simulink library "Control_System_Library"  (Simulink 8.0)
settings: Solver=ode45  StartTime=0.0  StopTime=10.0  RelTol=1e-3
values from neighbouring files (symbols this model uses):
  B_bias = [0 0 0]    [Initialize_UKF_Function.m]
  B_Init_Inertial = wrldmagm(Alt, Lat, Long, 2013)*1E-9    [Initialize_UKF_Function.m]
  I_c = [3.4 3.4 1.9]    [Initialize_UKF_Function.m]    (also in UKF_quaternion_withBias.m)
  NED_Init = dcmecef2ned(Lat, Long)*ECEF_Init    [Initialize_UKF_Function.m]
  q_i_s0 = init_attitude    [Initialize_UKF_Function.m]
  q_s_c = [1 0 0 0]    [Initialize_UKF_Function.m]    (also in Satellite2Controller_Conversion.m = dcm2quat(R); UKF_quaternion_withBias.m = [1; 0; 0; 0])
  Time_Start = 0    [Initialize_UKF_Function.m]
  Ts = .1    (= 0.1)    [Initialize_UKF_Function.m]
  w_bias = 0*[0.5 0.2 0.15]    [Initialize_UKF_Function.m]    (also in UKF_quaternion_withBias.m = zeros(3,1))
  w_init_s = [rand_w_x rand_w_y rand_w_z]    [Initialize_UKF_Function.m]
undefined symbols (not defined in the file or in its folder): aeroassertmsg, c, cd, DiscIntNeverNeededParam, dyear, Earth, epoch, fm, fn, k, maxdef, Newton, Raphson, sgp4, snorm, WGS84
libraries: commnoisgen2 x6, aerolibconvert2 x4, simulink x3, aerolibutil x2, aerolibtransform2 x2, dspmtrx3 x1, aerolibgravitysys x1
(part 1 of 3)
settings Model: Creator=bajackso  LastModifiedBy=nwford

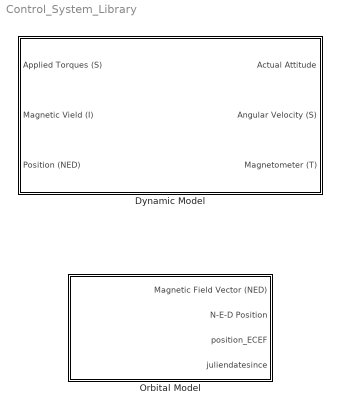
== system Control_System_Library ==
  Dynamic Model : Subsystem
  Orbital Model : Subsystem

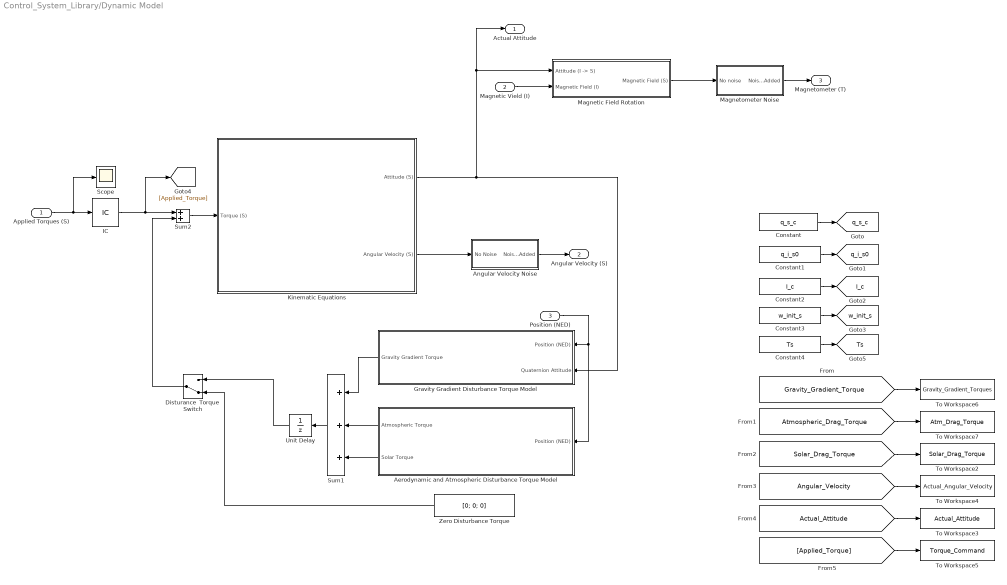
== system Control_System_Library/Dynamic Model ==
  Applied Torques (S) : Inport
  Magnetic Vield (I) : Inport  Port=2
  Position (NED) : Inport  Port=3
  Aerodynamic and Atmospheric Disturbance Torque Model : Subsystem
  Angular Velocity Noise : Subsystem
  Constant : Constant  Value=q_s_c
  Constant1 : Constant  Value=q_i_s0
  Constant2 : Constant  Value=I_c
  Constant3 : Constant  Value=w_init_s
  Constant4 : Constant  Value=Ts
  Disturance  Torque Switch : ManualSwitch  CurrentSetting=0
  Gravity Gradient Disturbance Torque Model : Subsystem
  IC : InitialCondition  Value=[0 0 0]
  Kinematic Equations : Subsystem
  Magnetic Field Rotation : Subsystem
  Magnetometer Noise : Subsystem
  Scope : Scope
      settings: TimeRange=10000
  Sum1 : Sum  Inputs=+++
  Sum2 : Sum
  To Workspace2 : ToWorkspace  VariableName=Solar_Drag_Torque  SampleTime=-1
      settings: Decimation=Decimation
  To Workspace3 : ToWorkspace  VariableName=Actual_Attitude  SampleTime=-1
      settings: Decimation=Decimation
  To Workspace4 : ToWorkspace  VariableName=Actual_Angular_Velocity  SampleTime=-1
      settings: Decimation=Decimation
  To Workspace5 : ToWorkspace  VariableName=Torque_Command  SampleTime=-1
      settings: Decimation=Decimation
  To Workspace6 : ToWorkspace  VariableName=Gravity_Gradient_Torques  SampleTime=-1
      settings: Decimation=Decimation
  To Workspace7 : ToWorkspace  VariableName=Atm_Drag_Torque  SampleTime=-1
      settings: Decimation=Decimation
  Unit Delay : UnitDelay  SampleTime=-1
  Zero Disturbance Torque : Constant  Value=[0; 0; 0]
  Actual Attitude : Outport
  Angular Velocity (S) : Outport  Port=2
  Magnetometer (T) : Outport  Port=3
  tag scope: I_c=global, Ts=global, q_i_s0=global, q_s_c=global, w_init_s=global
  wires:
  Unit Delay/1 -> Disturance  Torque Switch/1
  IC/1 -> [Applied_Torque], Sum2/1
  Kinematic Equations/1(Attitude (S)) -> Actual Attitude/1, Magnetic Field Rotation/1("Attitude (I -> S)"), Gravity Gradient Disturbance Torque Model/2(Quaternion Attitude)
  Applied Torques (S)/1 -> IC/1, Scope/1
  Sum2/1 -> Kinematic Equations/1(Torque (S))
  Sum1/1 -> Unit Delay/1
  Disturance  Torque Switch/1 -> Sum2/2
  Zero Disturbance Torque/1 -> Disturance  Torque Switch/2
  Position (NED)/1 -> Gravity Gradient Disturbance Torque Model/1(Position (NED)), Aerodynamic and Atmospheric Disturbance Torque Model/1(Position (NED))
  Gravity Gradient Disturbance Torque Model/1(Gravity Gradient Torque) -> Sum1/1
  Aerodynamic and Atmospheric Disturbance Torque Model/1(Atmospheric Torque) -> Sum1/2
  Aerodynamic and Atmospheric Disturbance Torque Model/2(Solar Torque) -> Sum1/3
  Angular Velocity Noise/1(Noise Added) -> Angular Velocity (S)/1
  Magnetometer Noise/1("Noise Added ") -> Magnetometer (T)/1
  Constant/1 -> [q_s_c]
  Constant1/1 -> [q_i_s0]
  Constant2/1 -> [I_c]
  Constant3/1 -> [w_init_s]
  Kinematic Equations/2(Angular Velocity (S)) -> Angular Velocity Noise/1(No Noise)
  Magnetic Vield (I)/1 -> Magnetic Field Rotation/2(Magnetic Field (I))
  Magnetic Field Rotation/1(Magnetic Field (S)) -> Magnetometer Noise/1(No noise)
  [Gravity_Gradient_Torque] -> To Workspace6/1
  [Atmospheric_Drag_Torque] -> To Workspace7/1
  [Solar_Drag_Torque] -> To Workspace2/1
  [Angular_Velocity] -> To Workspace4/1
  [Actual_Attitude] -> To Workspace3/1
  [Applied_Torque] -> To Workspace5/1
  Constant4/1 -> [Ts]

== system Control_System_Library/Orbital Model ==
  Constant : Constant  Value=Time_Start
  Digital Clock1 : DigitalClock  SampleTime=.1
  "JDepochdate " : Constant  Value=2456507.01579
  Rate Transition : RateTransition  X0=NED_Init
  Rate Transition1 : RateTransition  X0=B_Init_Inertial
  S2M : Gain  Gain=1/60
  SGP4 : MATLABFcn  MATLABFcn=sgp4(u(1))
  Subsystem : Subsystem
  Sum : Sum  Inputs=|++
  Sum1 : Sum  Inputs=|++
  gain : Gain  Gain=1/(60*24)
  km to m : Gain  Gain=1000
  Magnetic Field Vector (NED) : Outport  PortDimensions=3
  N-E-D Position : Outport  Port=2  PortDimensions=3
  position_ECEF : Outport  Port=3
  "juliendatesince " : Outport  Port=4  PortDimensions=1
  wires:
  Digital Clock1/1 -> S2M/1
  Subsystem/2(Position  (NED)) -> Rate Transition/1
  km to m/1 -> position_ECEF/1, Subsystem/1(Position  (ECEF))
  Subsystem/1(Magnetic Field  (NED)) -> Rate Transition1/1
  SGP4/1 -> km to m/1
  Rate Transition/1 -> N-E-D Position/1
  Rate Transition1/1 -> Magnetic Field Vector (NED)/1
  S2M/1 -> Sum/1
  Constant/1 -> Sum/2
  Sum/1 -> gain/1, SGP4/1
  "JDepochdate "/1 -> Sum1/1
  Sum1/1 -> "juliendatesince "/1
  gain/1 -> Sum1/2

== system Control_System_Library/Dynamic Model/Aerodynamic and Atmospheric Disturbance Torque Model ==
  Position (NED) : Inport
  MATLAB Function : MATLAB Function  TreatAsAtomicUnit=on
  MATLAB Function1 : MATLAB Function  TreatAsAtomicUnit=on
  Atmospheric Torque : Outport
  Solar Torque : Outport  Port=2
  tag scope: Atmospheric_Drag_Torque=global, Solar_Drag_Torque=global
  wires:
  MATLAB Function/1(ATM_Torque) -> [Atmospheric_Drag_Torque], Atmospheric Torque/1
  Position (NED)/1 -> MATLAB Function/1(R)
  MATLAB Function1/1(Solar_Torque) -> [Solar_Drag_Torque], Solar Torque/1

== system Control_System_Library/Dynamic Model/Angular Velocity Noise ==
  No Noise : Inport
  Manual Switch : ManualSwitch  CurrentSetting=0
  Mux : Mux  Inputs=3
  Sum : Sum  Inputs=|++
  X : commnoisgen2/Gaussian Noise Generator  m=w_bias(1)  d=gyro_noise  s=41  Ts=Ts  frameBased=off  sampPerFrame=1  orient=off  outDataType=double
  Y : commnoisgen2/Gaussian Noise Generator  m=w_bias(2)  d=gyro_noise  s=1235123  Ts=Ts  frameBased=off  sampPerFrame=1  orient=off  outDataType=double
  Z : commnoisgen2/Gaussian Noise Generator  m=w_bias(3)  d=gyro_noise  s=23523  Ts=Ts  frameBased=off  sampPerFrame=1  orient=off  outDataType=double
  Zero Noise : Constant  Value=0
  Noise Added : Outport
  wires:
  X/1 -> Mux/1
  Y/1 -> Mux/2
  Z/1 -> Mux/3
  No Noise/1 -> Sum/1
  Zero Noise/1 -> Manual Switch/2
  Mux/1 -> Manual Switch/1
  Sum/1 -> Noise Added/1
  Manual Switch/1 -> Sum/2

== system Control_System_Library/Dynamic Model/Gravity Gradient Disturbance Torque Model ==
  Position (NED) : Inport
  Quaternion Attitude : Inport  Port=2
  Conversion to Satellite Body Frame : aerolibutil/Quaternion Rotation
  MATLAB Function : MATLAB Function  TreatAsAtomicUnit=on
  Gravity Gradient Torque : Outport
  tag scope: Gravity_Gradient_Torque=global
  wires:
  MATLAB Function/1(G_grav) -> [Gravity_Gradient_Torque], Gravity Gradient Torque/1
  Quaternion Attitude/1 -> Conversion to Satellite Body Frame/1
  Position (NED)/1 -> Conversion to Satellite Body Frame/2
  Conversion to Satellite Body Frame/1 -> MATLAB Function/1(R)

== system Control_System_Library/Dynamic Model/Kinematic Equations ==
  Torque (S) : Inport
  Discrete-Time Integrator : DiscreteIntegrator  Commented=on  InitialConditionSource=external  InitialCondition=[0; 0; 0]  SampleTime=-1  ICPrevOutput=DiscIntNeverNeededParam  ICPrevScaledInput=DiscIntNeverNeededParam
  Discrete-Time Integrator1 : DiscreteIntegrator  Commented=on  InitialCondition=[0; 0; 0]  SampleTime=-1  ICPrevOutput=DiscIntNeverNeededParam  ICPrevScaledInput=DiscIntNeverNeededParam
  MATLAB Function : MATLAB Function  Commented=on  TreatAsAtomicUnit=on
  MATLAB Function1 : MATLAB Function  Commented=on  TreatAsAtomicUnit=on
  MATLAB Function2 : MATLAB Function  TreatAsAtomicUnit=on
  Matrix Multiply : Product  Commented=on  Multiplication=Matrix(*)
  Attitude (S) : Outport
  Angular Velocity (S) : Outport  Port=2
  tag scope: Actual_Attitude=global, Angular_Velocity=global
  wires:
  Discrete-Time Integrator/1 -> Matrix Multiply/2, MATLAB Function/3(w)
  MATLAB Function/1(w_dot) -> Discrete-Time Integrator/1
  Matrix Multiply/1 -> Discrete-Time Integrator1/1
  Discrete-Time Integrator1/1 -> MATLAB Function1/1(EA)
  MATLAB Function1/1(B) -> Matrix Multiply/1
  Torque (S)/1 -> MATLAB Function2/3(Torque_s)
  [I_c] -> MATLAB Function2/1(I_c)
  [q_i_s0] -> MATLAB Function2/4(q0_i_s)
  MATLAB Function2/1(w_s) -> [Angular_Velocity], Angular Velocity (S)/1
  MATLAB Function2/2(q_i_s) -> [Actual_Attitude], Attitude (S)/1
  [w_init_s] -> MATLAB Function2/2(w_init_s)
  [q_s_c] -> MATLAB Function2/5(q_s_c)
  [Ts] -> MATLAB Function2/6(Ts)

== system Control_System_Library/Dynamic Model/Magnetic Field Rotation ==
  "Attitude (I -> S)" : Inport
  Magnetic Field (I) : Inport  Port=2
  IC : InitialCondition  Value=q_i_s0
  IC1 : InitialCondition  Value=B_Init_Inertial
  Quaternion Rotation1 : aerolibutil/Quaternion Rotation
  Transpose1 : dspmtrx3/Transpose  Hermitian=off  overflowFlag=off
  Magnetic Field (S) : Outport
  wires:
  Quaternion Rotation1/1 -> Magnetic Field (S)/1
  Magnetic Field (I)/1 -> IC1/1
  Transpose1/1 -> Quaternion Rotation1/1
  "Attitude (I -> S)"/1 -> IC/1
  IC/1 -> Transpose1/1
  IC1/1 -> Quaternion Rotation1/2

== system Control_System_Library/Dynamic Model/Magnetometer Noise ==
  No noise : Inport
  Manual Switch : ManualSwitch
  Mux : Mux  Inputs=3
  Sum : Sum  Inputs=|++
  X : commnoisgen2/Gaussian Noise Generator  m=B_bias(1)  d=B_noise  s=2341  Ts=Ts  frameBased=off  sampPerFrame=1  orient=off  outDataType=double
  Y : commnoisgen2/Gaussian Noise Generator  m=B_bias(2)  d=B_noise  s=64236  Ts=Ts  frameBased=off  sampPerFrame=1  orient=off  outDataType=double
  Z : commnoisgen2/Gaussian Noise Generator  m=B_bias(3)  d=B_noise  s=346312  Ts=Ts  frameBased=off  sampPerFrame=1  orient=off  outDataType=double
  Zero Noise : Constant  Value=0
  "Noise Added " : Outport
  wires:
  X/1 -> Mux/1
  Y/1 -> Mux/2
  Z/1 -> Mux/3
  Mux/1 -> Manual Switch/1
  Zero Noise/1 -> Manual Switch/2
  Manual Switch/1 -> Sum/2
  No noise/1 -> Sum/1
  Sum/1 -> "Noise Added "/1

== system Control_System_Library/Orbital Model/Subsystem ==
  Position  (ECEF) : Inport
  Demux : Demux  Outputs=2
  Direction Cosine Matrix ECEF to NED : aerolibtransform2/Direction Cosine Matrix ECEF to NED
  ECEF Position to LLA1 : aerolibtransform2/ECEF Position to LLA  units=Metric (MKS)  ptype=Earth (WGS84)  F=1/298.257223563  R=6378137
  Gain : Gain  Gain=1E-9
  Matrix Multiply : Product  Multiplication=Matrix(*)
  World Magnetic Model 2010 : Subsystem  AncestorBlock=aerolibgravity2/World Magnetic Model 2010  mask(World Magnetic Model 2010){units=Metric (MKS), time_in=off, month=January, day=1, year=2010, action=Error, h_out=off, dec_out=off, inc_out=off, ti_out=off}
      mask prompts: time_in "Input decimal year"; action "Action for out of range input:"; h_out "Output horizontal intensity"; dec_out "Output declination"; inc_out "Output inclination"; ti_out "Output total intensity"
      mask help:
      | Calculate the Earth's magnetic field at a specific location and time using the World Magnetic Model (WMM). This model is valid for the year 2010 through the year 2015.
      |
      | The WMM-2010 can be found on the web at http://www.ngdc.noaa.gov/geomag/WMM/DoDWMM.shtml and in "NOAA Technical Report: The US/UK World Magnetic Model for 2010-2015 ".
      |
      | Height is entered in length units of selected unit system. Latitude and longitude are entered in degrees.
      mask init:
      | [ports,dyear,maxdef,epoch,c,cd,fn,fm,snorm,k]=aeroicon('aeroblkwmm2010','icon');
      mask Help: eval('asbhelp');
      mask TypeOptions units: Metric (MKS) | English
      mask Callback time_in: aeroicon('aeroblkwmm');
      mask TypeOptions month: January | February | March | April | May | June | July | August | September | October | November | December
      mask Callback month: aeroicon('aeroblkwmm');
      mask TypeOptions day: 1 | 2 | 3 | 4 | 5 | 6 | 7 | 8 | 9 | 10 | 11 | 12 | 13 | 14 | 15 | 16 | 17 | 18 | 19 | 20 | 21 | 22 | 23 | 24 | 25 | 26 | 27 | 28 | 29 | 30 | 31
      mask Callback day: aeroicon('aeroblkwmm');
      mask TypeOptions year: 2010 | 2011 | 2012 | 2013 | 2014 | 2015
      mask Callback year: aeroicon('aeroblkwmm');
      mask TypeOptions action: None | Warning | Error
      mask Display:
      | port_label(ports(1).type,ports(1).port,ports(1).txt);
      | port_label(ports(2).type,ports(2).port,ports(2).txt,'texmode','on');
      | port_label(ports(3).type,ports(3).port,ports(3).txt,'texmode','on');
      | port_label(ports(4).type,ports(4).port,ports(4).txt);
      | port_label(ports(5).type,ports(5).port,ports(5).txt);
      | port_label(ports(6).type,ports(6).port,ports(6).txt);
      | port_label(ports(7).type,ports(7).port,ports(7).txt);
      | port_label(ports(8).type,ports(8).port,ports(8).txt);
      | port_label(ports(9).type,ports(9).port,ports(9).txt);
  Magnetic Field  (NED) : Outport
  Position  (NED) : Outport  Port=2
  wires:
  World Magnetic Model 2010/1(Magnetic Field) -> Gain/1
  Gain/1 -> Magnetic Field  (NED)/1
  Position  (ECEF)/1 -> ECEF Position to LLA1/1, Matrix Multiply/2
  ECEF Position to LLA1/2 -> World Magnetic Model 2010/1(Altitude)
  Demux/1 -> World Magnetic Model 2010/2(Latitude)
  Demux/2 -> World Magnetic Model 2010/3(Longitude)
  ECEF Position to LLA1/1 -> Demux/1, Direction Cosine Matrix ECEF to NED/1
  Direction Cosine Matrix ECEF to NED/1 -> Matrix Multiply/1
  Matrix Multiply/1 -> Position  (NED)/1

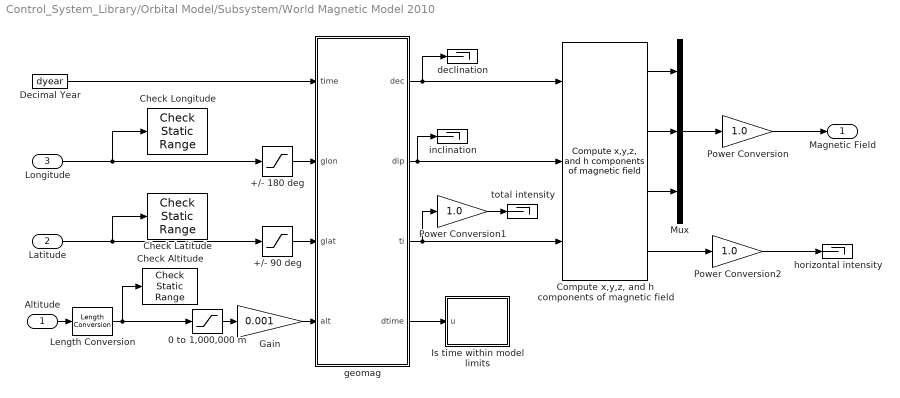
== system Control_System_Library/Orbital Model/Subsystem/World Magnetic Model 2010 ==
  Altitude : Inport
  Latitude : Inport  Port=2
  Longitude : Inport  Port=3
  +/- 180 deg : Saturate  UpperLimit=180.0  LowerLimit=-180.0
  +/- 90 deg : Saturate  UpperLimit=90.0  LowerLimit=-90.0
  0 to 1,000,000 m : Saturate  UpperLimit=1000000.0  LowerLimit=0
  Check Altitude : simulink/Model Verification/Check  Static Range  Description=0 <= u <= 1000000  max=1000000  max_included=on  min=0  min_included=on  enabled=on  callback=aeroassertmsg('aeroblkwmm','alt','error')  stopWhenAssertionFail=on  export=off  icon=graphic
  Check Latitude : simulink/Model Verification/Check  Static Range  Description=-90 <= u <= 90  max=90  max_included=on  min=-90  min_included=on  enabled=on  callback=aeroassertmsg('aeroblkwmm','lat','error')  stopWhenAssertionFail=on  export=off  icon=graphic
  Check Longitude : simulink/Model Verification/Check  Static Range  Description=-180 <= u <= 180  max=180  max_included=on  min=-180  min_included=on  enabled=on  callback=aeroassertmsg('aeroblkwmm','lon','error')  stopWhenAssertionFail=on  export=off  icon=graphic
  "Compute x,y,z, and h components of magnetic field" : aerolibgravitysys/Compute x,y,z, and h components of magnetic field
  Decimal Year : Constant  Value=dyear  OutDataTypeStr=Inherit: Inherit via back propagation
  Gain : Gain  Gain=0.001  SaturateOnIntegerOverflow=on  OutDataTypeStr=Inherit: Same as input  ParamDataTypeStr=Inherit: Same as input
  Is time within model limits : Subsystem  Description=0 <= u <= 5  mask(Checks_SRange){max=5, max_included=on, min=0, min_included=on, enabled=on, callback=aeroassertmsg('aeroblkwmm','time','error'), stopWhenAssertionFail=on, export=off, icon=graphic}
      mask prompts: max "Upper bound:"; max_included "Inclusive upper bound"; min "Lower bound:"; min_included "Inclusive lower bound"; enabled "Enable assertion"; callback "Simulation callback when assertion fails (optional):"; stopWhenAssertionFail "Stop simulation when assertion fails"; export "Output assertion signal"; icon "Select icon type:"
      mask help: Assert that the input signal lies between a static lower and upper bound or optionally equals either bound.
      mask init:
      | update_assert_sys(gcbh);
      mask TypeOptions icon: graphic | text
      mask Display: image(imread('Checks_SRange.bmp','bmp'),'center')
  Length Conversion : aerolibconvert2/Length Conversion  IU=m  OU=m
  Mux : Mux  Inputs=3
  Power Conversion : Gain  Gain=1.0  SaturateOnIntegerOverflow=on  OutDataTypeStr=Inherit: Same as input  ParamDataTypeStr=Inherit: Same as input
  Power Conversion1 : Gain  Gain=1.0  SaturateOnIntegerOverflow=on  OutDataTypeStr=Inherit: Same as input  ParamDataTypeStr=Inherit: Same as input
  Power Conversion2 : Gain  Gain=1.0  SaturateOnIntegerOverflow=on  OutDataTypeStr=Inherit: Same as input  ParamDataTypeStr=Inherit: Same as input
  declination : Terminator
  geomag : Subsystem  AncestorBlock=aerolibgravitysys/geomag
  horizontal intensity : Terminator
  inclination : Terminator
  total intensity : Terminator
  Magnetic Field : Outport
  wires:
  geomag/4(dtime) -> Is time within model limits/1(u)
  0 to 1,000,000 m/1 -> Gain/1
  +/- 180 deg/1 -> geomag/2(glon)
  +/- 90 deg/1 -> geomag/3(glat)
  Power Conversion2/1 -> horizontal intensity/1
  Power Conversion1/1 -> total intensity/1
  Power Conversion/1 -> Magnetic Field/1
  Mux/1 -> Power Conversion/1
  geomag/1(dec) -> declination/1, "Compute x,y,z, and h components of magnetic field"/1
  Gain/1 -> geomag/4(alt)
  Longitude/1 -> Check Longitude/1, +/- 180 deg/1
  Latitude/1 -> Check Latitude/1, +/- 90 deg/1
  geomag/3(ti) -> Power Conversion1/1, "Compute x,y,z, and h components of magnetic field"/3
  geomag/2(dip) -> inclination/1, "Compute x,y,z, and h components of magnetic field"/2
  Decimal Year/1 -> geomag/1(time)
  "Compute x,y,z, and h components of magnetic field"/4 -> Power Conversion2/1
  "Compute x,y,z, and h components of magnetic field"/3 -> Mux/3
  "Compute x,y,z, and h components of magnetic field"/2 -> Mux/2
  "Compute x,y,z, and h components of magnetic field"/1 -> Mux/1
  Length Conversion/1 -> Check Altitude/1, 0 to 1,000,000 m/1
  Altitude/1 -> Length Conversion/1

== system Control_System_Library/Orbital Model/Subsystem/World Magnetic Model 2010/Is time within model limits ==
  u : Inport
  Assertion : Assertion  Enabled=on  AssertionFailFcn=evalin('base',callback)
  conjunction : Logic
  max_relop : RelationalOperator  Operator=<=  InputSameDT=on
  max_val : Constant  Value=max
  maxtype : DataTypeConversion  SaturateOnIntegerOverflow=on  RndMeth=Zero
  min_relop : RelationalOperator  Operator=<=  InputSameDT=on
  min_val : Constant  Value=min
  mintype : DataTypeConversion  SaturateOnIntegerOverflow=on  RndMeth=Zero
  out : Terminator
  wires:
  u/1 -> min_relop/2, max_relop/1
  min_val/1 -> mintype/1
  max_val/1 -> maxtype/1
  min_relop/1 -> conjunction/1
  max_relop/1 -> conjunction/2
  conjunction/1 -> out/1, Assertion/1
  mintype/1 -> min_relop/1
  maxtype/1 -> max_relop/2

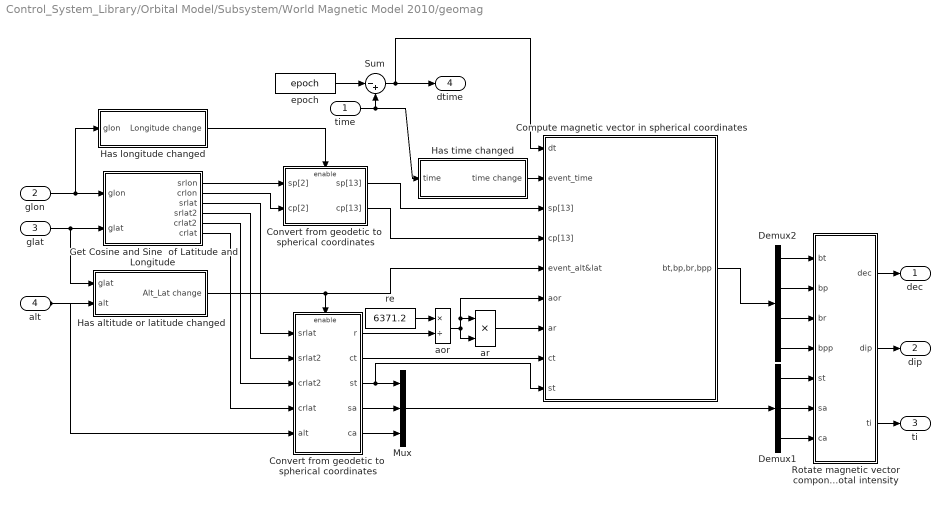
== system Control_System_Library/Orbital Model/Subsystem/World Magnetic Model 2010/geomag ==
  time : Inport
  glon : Inport  Port=2
  glat : Inport  Port=3
  alt : Inport  Port=4
  Compute magnetic vector in spherical coordinates : Subsystem  TreatAsAtomicUnit=on
  Convert from geodetic to  spherical coordinates : Subsystem  TreatAsAtomicUnit=on
  "Convert from geodetic to  spherical coordinates " : Subsystem
  Demux1 : Demux  Outputs=3
  Demux2 : Demux
  Get Cosine and Sine  of Latitude and Longitude : Subsystem
  Has altitude or latitude changed : Subsystem
  "Has longitude changed " : Subsystem
  Has time changed : Subsystem
  Mux : Mux  Inputs=3
  "Rotate magnetic vector components  to geodetic from spherical and  compute declination, inclination  and total intensity" : Subsystem
  Sum : Sum  Inputs=|-+  SaturateOnIntegerOverflow=on
  aor : Product  Inputs=*/  SaturateOnIntegerOverflow=on  OutDataTypeStr=Inherit: Same as first input
  ar : Product  SaturateOnIntegerOverflow=on  OutDataTypeStr=Inherit: Same as first input
  epoch : Constant  Value=epoch  OutDataTypeStr=Inherit: Inherit via back propagation
  re : Constant  Value=6371.2  OutDataTypeStr=Inherit: Inherit via back propagation
  dec : Outport
  dip : Outport  Port=2
  ti : Outport  Port=3
  dtime : Outport  Port=4
  wires:
  Demux2/3 -> "Rotate magnetic vector components  to geodetic from spherical and  compute declination, inclination  and total intensity"/3(br)
  Demux2/2 -> "Rotate magnetic vector components  to geodetic from spherical and  compute declination, inclination  and total intensity"/2(bp)
  Compute magnetic vector in spherical coordinates/1(bt,bp,br,bpp) -> Demux2/1
  Demux1/3 -> "Rotate magnetic vector components  to geodetic from spherical and  compute declination, inclination  and total intensity"/7(ca)
  Demux1/2 -> "Rotate magnetic vector components  to geodetic from spherical and  compute declination, inclination  and total intensity"/6(sa)
  Demux1/1 -> "Rotate magnetic vector components  to geodetic from spherical and  compute declination, inclination  and total intensity"/5(st)
  Demux2/4 -> "Rotate magnetic vector components  to geodetic from spherical and  compute declination, inclination  and total intensity"/4(bpp)
  Demux2/1 -> "Rotate magnetic vector components  to geodetic from spherical and  compute declination, inclination  and total intensity"/1(bt)
  Mux/1 -> Demux1/1
  Convert from geodetic to  spherical coordinates/5(ca) -> Mux/3
  Convert from geodetic to  spherical coordinates/4(sa) -> Mux/2
  Convert from geodetic to  spherical coordinates/3(st) -> Compute magnetic vector in spherical coordinates/9(st), Mux/1
  epoch/1 -> Sum/1
  Convert from geodetic to  spherical coordinates/2(ct) -> Compute magnetic vector in spherical coordinates/8(ct)
  Get Cosine and Sine  of Latitude and Longitude/6(crlat) -> Convert from geodetic to  spherical coordinates/4(crlat)
  Get Cosine and Sine  of Latitude and Longitude/3(srlat) -> Convert from geodetic to  spherical coordinates/1(srlat)
  "Rotate magnetic vector components  to geodetic from spherical and  compute declination, inclination  and total intensity"/3(ti) -> ti/1
  "Rotate magnetic vector components  to geodetic from spherical and  compute declination, inclination  and total intensity"/2(dip) -> dip/1
  "Rotate magnetic vector components  to geodetic from spherical and  compute declination, inclination  and total intensity"/1(dec) -> dec/1
  ar/1 -> Compute magnetic vector in spherical coordinates/7(ar)
  re/1 -> aor/1
  Convert from geodetic to  spherical coordinates/1(r) -> aor/2
  aor/1 -> ar/1, Compute magnetic vector in spherical coordinates/6(aor), ar/2
  "Convert from geodetic to  spherical coordinates "/2(cp[13]) -> Compute magnetic vector in spherical coordinates/4(cp[13])
  "Convert from geodetic to  spherical coordinates "/1(sp[13]) -> Compute magnetic vector in spherical coordinates/3(sp[13])
  Has altitude or latitude changed/1(Alt_Lat change) -> Compute magnetic vector in spherical coordinates/5(event_alt&lat), Convert from geodetic to  spherical coordinates/Enable
  Get Cosine and Sine  of Latitude and Longitude/5(crlat2) -> Convert from geodetic to  spherical coordinates/3(crlat2)
  Get Cosine and Sine  of Latitude and Longitude/4(srlat2) -> Convert from geodetic to  spherical coordinates/2(srlat2)
  Get Cosine and Sine  of Latitude and Longitude/2(crlon) -> "Convert from geodetic to  spherical coordinates "/2(cp[2])
  Get Cosine and Sine  of Latitude and Longitude/1(srlon) -> "Convert from geodetic to  spherical coordinates "/1(sp[2])
  alt/1 -> Convert from geodetic to  spherical coordinates/5(alt), Has altitude or latitude changed/2(alt)
  glat/1 -> Get Cosine and Sine  of Latitude and Longitude/2(glat), Has altitude or latitude changed/1(glat)
  glon/1 -> Get Cosine and Sine  of Latitude and Longitude/1(glon), "Has longitude changed "/1(glon)
  "Has longitude changed "/1(Longitude change) -> "Convert from geodetic to  spherical coordinates "/Enable
  Has time changed/1(time change) -> Compute magnetic vector in spherical coordinates/2(event_time)
  time/1 -> Sum/2, Has time changed/1(time)
  Sum/1 -> dtime/1, Compute magnetic vector in spherical coordinates/1(dt)

== system Control_System_Library/Orbital Model/Subsystem/World Magnetic Model 2010/geomag/Compute magnetic vector in spherical coordinates ==
  dt : Inport
  event_time : Inport  Port=2
  sp[13] : Inport  Port=3
  cp[13] : Inport  Port=4
  event_alt&lat : Inport  Port=5
  aor : Inport  Port=6
  ar : Inport  Port=7
  ct : Inport  Port=8
  st : Inport  Port=9
  Constant : Constant  OutDataTypeStr=Inherit: Inherit via back propagation
  For Iterator : ForIterator  ResetStates=reset  IterationLimit=maxdef
  For Iterator Subsystem : Subsystem  TreatAsAtomicUnit=on
  Mux : Mux
  Product8 : Product  SaturateOnIntegerOverflow=on  OutDataTypeStr=Inherit: Same as first input
  Sum : Sum  Inputs=++|  SaturateOnIntegerOverflow=on
  Sum1 : Sum  Inputs=++|  SaturateOnIntegerOverflow=on
  Unit Delay : UnitDelay  SampleTime=-1
  Unit Delay2 : UnitDelay  InitialCondition=[0 0 0 0]  SampleTime=-1
  ar(n) : Switch  Criteria=u2 > Threshold  Threshold=1  SaturateOnIntegerOverflow=on
  bt,bp,br,bpp : Outport
  wires:
  Sum1/1 -> Unit Delay2/1, bt,bp,br,bpp/1
  Unit Delay2/1 -> Sum1/1
  Mux/1 -> Sum1/2
  For Iterator Subsystem/4(bpp) -> Mux/4
  For Iterator Subsystem/3(br) -> Mux/3
  For Iterator Subsystem/2(bp) -> Mux/2
  For Iterator Subsystem/1(bt) -> Mux/1
  dt/1 -> For Iterator Subsystem/10(dt)
  cp[13]/1 -> For Iterator Subsystem/9(cp)
  sp[13]/1 -> For Iterator Subsystem/8(sp)
  st/1 -> For Iterator Subsystem/7(st)
  ct/1 -> For Iterator Subsystem/6(ct)
  Constant/1 -> Sum/2
  Sum/1 -> For Iterator Subsystem/3(D4)
  ar(n)/1 -> Product8/1
  Product8/1 -> For Iterator Subsystem/1(ar), Unit Delay/1
  Unit Delay/1 -> ar(n)/1
  aor/1 -> Product8/2
  event_time/1 -> For Iterator Subsystem/5(event_time)
  ar/1 -> ar(n)/3
  event_alt&lat/1 -> For Iterator Subsystem/4(event_alt&lat)
  For Iterator/1 -> Sum/1, For Iterator Subsystem/2(n), ar(n)/2

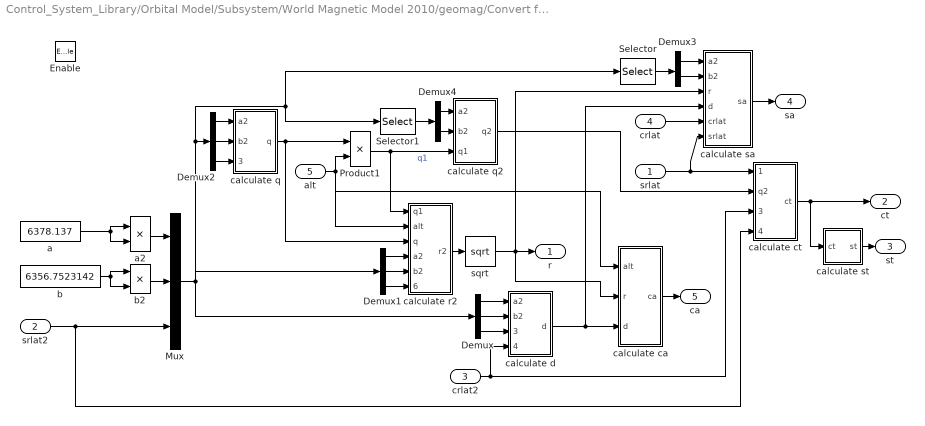
== system Control_System_Library/Orbital Model/Subsystem/World Magnetic Model 2010/geomag/Convert from geodetic to  spherical coordinates ==
  srlat : Inport
  srlat2 : Inport  Port=2
  crlat2 : Inport  Port=3
  crlat : Inport  Port=4
  alt : Inport  Port=5
  Enable : EnablePort  PropagateVarSize=During execution
  Demux : Demux  Outputs=3
  Demux1 : Demux  Outputs=3
  Demux2 : Demux  Outputs=3
  Demux3 : Demux  Outputs=2
  Demux4 : Demux  Outputs=2
  Mux : Mux  Inputs=3
  Product1 : Product  SaturateOnIntegerOverflow=on  OutDataTypeStr=Inherit: Same as first input
  Selector : Selector  InputPortWidth=3  IndexOptions=Index vector (dialog)  Indices=[1 2]  OutputSizes=1
  Selector1 : Selector  InputPortWidth=3  IndexOptions=Index vector (dialog)  Indices=[1 2]  OutputSizes=1
  a : Constant  Value=6378.137  OutDataTypeStr=Inherit: Inherit via back propagation
  a2 : Product  SaturateOnIntegerOverflow=on  OutDataTypeStr=Inherit: Same as first input
  b : Constant  Value=6356.7523142  OutDataTypeStr=Inherit: Inherit via back propagation
  b2 : Product  SaturateOnIntegerOverflow=on  OutDataTypeStr=Inherit: Same as first input
  calculate ca : Subsystem
  calculate ct : Subsystem
  calculate d : Subsystem
  calculate q : Subsystem
  calculate q2 : Subsystem
  calculate r2 : Subsystem
  calculate sa : Subsystem
  calculate st : Subsystem
  sqrt : Sqrt  AlgorithmType=Newton-Raphson  SaturateOnIntegerOverflow=on
  r : Outport
  ct : Outport  Port=2
  st : Outport  Port=3
  sa : Outport  Port=4
  ca : Outport  Port=5
  wires:
  Demux/3 -> calculate d/3(srlat2)
  Demux4/2 -> calculate q2/2(b2)
  Demux4/1 -> calculate q2/1(a2)
  Selector1/1 -> Demux4/1
  Selector/1 -> Demux3/1
  Demux3/2 -> calculate sa/2(b2)
  Demux3/1 -> calculate sa/1(a2)
  Mux/1 -> Selector/1, Selector1/1, Demux2/1, Demux/1, Demux1/1
  Demux2/3 -> calculate q/3(srlat2)
  Demux2/2 -> calculate q/2(b2)
  Demux2/1 -> calculate q/1(a2)
  Demux1/3 -> calculate r2/6(srlat2)
  Demux1/2 -> calculate r2/5(b2)
  Demux1/1 -> calculate r2/4(a2)
  Demux/1 -> calculate d/1(a2)
  Demux/2 -> calculate d/2(b2)
  calculate q2/1(q2) -> calculate ct/2(q2)
  b2/1 -> Mux/2
  b/1 -> b2/1, b2/2
  a2/1 -> Mux/1
  a/1 -> a2/1, a2/2
  calculate sa/1(sa) -> sa/1
  crlat/1 -> calculate sa/5(crlat)
  calculate ca/1(ca) -> ca/1
  calculate d/1(d) -> calculate sa/4(d), calculate ca/3(d)
  sqrt/1 -> calculate ca/2(r), calculate sa/3(r), r/1
  calculate r2/1(r2) -> sqrt/1
  calculate st/1(st) -> st/1
  calculate ct/1(ct) -> calculate st/1(ct), ct/1
  srlat/1 -> calculate sa/6(srlat), calculate ct/1(srlat)
  crlat2/1 -> calculate ct/3(crlat2), calculate d/4(crlat2)
  alt/1 -> calculate r2/2(alt), calculate ca/1(alt), Product1/2
  Product1/1 -> calculate r2/1(q1), calculate q2/3(q1)  "q1"
  calculate q/1(q) -> calculate r2/3(q), Product1/1
  srlat2/1 -> Mux/3, calculate ct/4(srlat2)

== system Control_System_Library/Orbital Model/Subsystem/World Magnetic Model 2010/geomag/Convert from geodetic to  spherical coordinates  ==
  sp[2] : Inport
  cp[2] : Inport  Port=2
  Enable : EnablePort  PropagateVarSize=During execution
  For Iterator Subsystem : Subsystem  TreatAsAtomicUnit=on
  Mux : Mux  Inputs=3
  Mux1 : Mux  Inputs=3
  cp[1] : Constant  OutDataTypeStr=Inherit: Inherit via back propagation
  sp[1] : Constant  Value=0  OutDataTypeStr=Inherit: Inherit via back propagation
  sp[13] : Outport  InitialOutput=[ zeros(1,13) ]
  cp[13] : Outport  Port=2  InitialOutput=[ zeros(1,13) ]
  wires:
  sp[1]/1 -> Mux1/1
  cp[1]/1 -> Mux/1
  Mux/1 -> cp[13]/1
  For Iterator Subsystem/2(cp[11]) -> Mux/3
  For Iterator Subsystem/1(sp[11]) -> Mux1/3
  cp[2]/1 -> For Iterator Subsystem/2(cp[2]), Mux/2
  sp[2]/1 -> For Iterator Subsystem/1(sp[2]), Mux1/2
  Mux1/1 -> sp[13]/1

== system Control_System_Library/Orbital Model/Subsystem/World Magnetic Model 2010/geomag/Get Cosine and Sine  of Latitude and Longitude ==
  glon : Inport
  glat : Inport  Port=2
  Angle Conversion : aerolibconvert2/Angle Conversion  IU=deg  OU=rad
  Demux : Demux  Outputs=2
  Demux1 : Demux  Outputs=2
  Mux : Mux  Inputs=2
  Product : Product  SaturateOnIntegerOverflow=on  OutDataTypeStr=Inherit: Same as first input
  Product1 : Product  SaturateOnIntegerOverflow=on  OutDataTypeStr=Inherit: Same as first input
  sincos : Trigonometry  Operator=sincos
  srlon : Outport
  crlon : Outport  Port=2
  srlat : Outport  Port=3
  srlat2 : Outport  Port=4
  crlat2 : Outport  Port=5
  crlat : Outport  Port=6
  wires:
  Demux1/2 -> Product1/2, Product1/1, crlat/1
  Demux/2 -> Product/2, Product/1, srlat/1
  Product1/1 -> crlat2/1
  Product/1 -> srlat2/1
  Demux1/1 -> crlon/1
  Demux/1 -> srlon/1
  glat/1 -> Mux/2
  glon/1 -> Mux/1
  sincos/2 -> Demux1/1
  sincos/1 -> Demux/1
  Mux/1 -> Angle Conversion/1
  Angle Conversion/1 -> sincos/1

== system Control_System_Library/Orbital Model/Subsystem/World Magnetic Model 2010/geomag/Has altitude or latitude changed ==
  glat : Inport
  alt : Inport  Port=2
  Logical Operator : Logic  Operator=OR  AllPortsSameDT=off
  Relational Operator : RelationalOperator  Operator=~=
  Relational Operator1 : RelationalOperator  Operator=~=
  oalt : Memory  X0=-1000  InheritSampleTime=on
  olat : Memory  X0=-1000  InheritSampleTime=on
  Alt_Lat change : Outport
  wires:
  Logical Operator/1 -> Alt_Lat change/1
  glat/1 -> olat/1, Relational Operator/1
  Relational Operator1/1 -> Logical Operator/2
  Relational Operator/1 -> Logical Operator/1
  oalt/1 -> Relational Operator1/2
  olat/1 -> Relational Operator/2
  alt/1 -> oalt/1, Relational Operator1/1

== system Control_System_Library/Orbital Model/Subsystem/World Magnetic Model 2010/geomag/Has longitude changed  ==
  glon : Inport
  Relational Operator : RelationalOperator  Operator=~=
  olon : Memory  X0=-1000  InheritSampleTime=on
  Longitude change : Outport
  wires:
  Relational Operator/1 -> Longitude change/1
  glon/1 -> olon/1, Relational Operator/1
  olon/1 -> Relational Operator/2

== system Control_System_Library/Orbital Model/Subsystem/World Magnetic Model 2010/geomag/Has time changed ==
  time : Inport
  Relational Operator : RelationalOperator  Operator=~=
  otime : Memory  X0=-1000  InheritSampleTime=on
  time change : Outport
  wires:
  otime/1 -> Relational Operator/2
  time/1 -> Relational Operator/1, otime/1
  Relational Operator/1 -> time change/1

== system Control_System_Library/Orbital Model/Subsystem/World Magnetic Model 2010/geomag/Rotate magnetic vector components  to geodetic from spherical and  compute declination, inclination  and total intensity ==
  bt : Inport
  bp : Inport  Port=2
  br : Inport  Port=3
  bpp : Inport  Port=4
  st : Inport  Port=5
  sa : Inport  Port=6
  ca : Inport  Port=7
  Calculate bx : Subsystem
  Calculate by : Subsystem
  Calculate bz : Subsystem
  "Compute declination, inclination,  and total intensity" : Subsystem
  Demux : Demux
  Demux1 : Demux
  Mux : Mux
  dec : Outport
  dip : Outport  Port=2
  ti : Outport  Port=3
  wires:
  "Compute declination, inclination,  and total intensity"/2(dip) -> dip/1
  "Compute declination, inclination,  and total intensity"/1(dec) -> dec/1
  Calculate bz/1(bz) -> "Compute declination, inclination,  and total intensity"/3(bz)
  Calculate bx/1(bx) -> "Compute declination, inclination,  and total intensity"/2(bx)
  Calculate by/1(by) -> "Compute declination, inclination,  and total intensity"/1(by)
  "Compute declination, inclination,  and total intensity"/3(ti) -> ti/1
  Demux1/4 -> Calculate bz/4(br)
  Demux1/3 -> Calculate bz/3(bt)
  Demux1/2 -> Calculate bz/2(sa)
  Demux1/1 -> Calculate bz/1(ca)
  Mux/1 -> Demux1/1, Demux/1
  Demux/4 -> Calculate bx/4(br)
  Demux/3 -> Calculate bx/3(bt)
  Demux/2 -> Calculate bx/2(sa)
  Demux/1 -> Calculate bx/1(ca)
  br/1 -> Mux/4
  bt/1 -> Mux/3
  sa/1 -> Mux/2
  ca/1 -> Mux/1
  bp/1 -> Calculate by/1(bp)
  bpp/1 -> Calculate by/3(bpp)
  st/1 -> Calculate by/2(st)

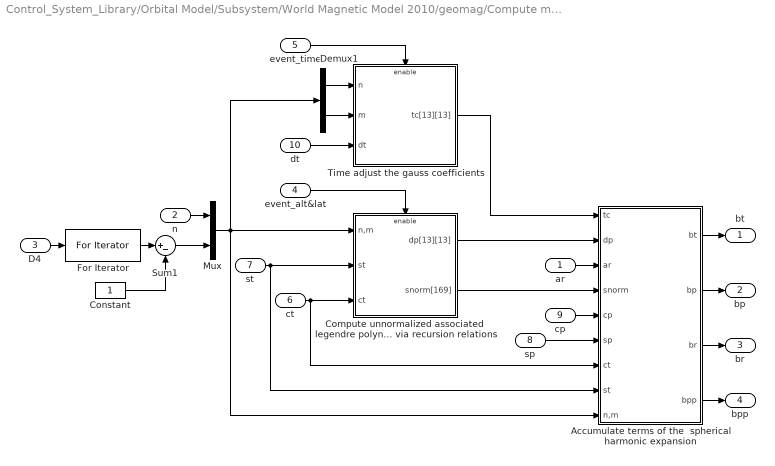
== system Control_System_Library/Orbital Model/Subsystem/World Magnetic Model 2010/geomag/Compute magnetic vector in spherical coordinates/For Iterator Subsystem ==
  ar : Inport
  n : Inport  Port=2
  D4 : Inport  Port=3
  event_alt&lat : Inport  Port=4
  event_time : Inport  Port=5
  ct : Inport  Port=6
  st : Inport  Port=7
  sp : Inport  Port=8
  cp : Inport  Port=9
  dt : Inport  Port=10
  Accumulate terms of the  spherical harmonic expansion : Subsystem
  Compute unnormalized associated  legendre polynomials and  derivatives via recursion relations : Subsystem  TreatAsAtomicUnit=on
  Constant : Constant  OutDataTypeStr=Inherit: Inherit via back propagation
  Demux1 : Demux  Outputs=2
  For Iterator : ForIterator  ResetStates=reset  IterationSource=external  IterationLimit=maxdef
  Mux : Mux  Inputs=2
  Sum1 : Sum  Inputs=|+-  SaturateOnIntegerOverflow=on  OutDataTypeStr=Inherit: Same as first input
  Time adjust the gauss coefficients : Subsystem  TreatAsAtomicUnit=on
  bt : Outport
  bp : Outport  Port=2
  br : Outport  Port=3
  bpp : Outport  Port=4
  wires:
  Accumulate terms of the  spherical harmonic expansion/4(bpp) -> bpp/1
  Sum1/1 -> Mux/2
  For Iterator/1 -> Sum1/1
  Demux1/2 -> Time adjust the gauss coefficients/2(m)
  Demux1/1 -> Time adjust the gauss coefficients/1(n)
  n/1 -> Mux/1
  Mux/1 -> Accumulate terms of the  spherical harmonic expansion/9(n,m), Compute unnormalized associated  legendre polynomials and  derivatives via recursion relations/1(n,m), Demux1/1
  Time adjust the gauss coefficients/1(tc[13][13]) -> Accumulate terms of the  spherical harmonic expansion/1(tc)
  ar/1 -> Accumulate terms of the  spherical harmonic expansion/3(ar)
  Accumulate terms of the  spherical harmonic expansion/2(bp) -> bp/1
  Accumulate terms of the  spherical harmonic expansion/1(bt) -> bt/1
  Accumulate terms of the  spherical harmonic expansion/3(br) -> br/1
  Compute unnormalized associated  legendre polynomials and  derivatives via recursion relations/1(dp[13][13]) -> Accumulate terms of the  spherical harmonic expansion/2(dp)
  Compute unnormalized associated  legendre polynomials and  derivatives via recursion relations/2(snorm[169]) -> Accumulate terms of the  spherical harmonic expansion/4(snorm)
  sp/1 -> Accumulate terms of the  spherical harmonic expansion/6(sp)
  cp/1 -> Accumulate terms of the  spherical harmonic expansion/5(cp)
  ct/1 -> Accumulate terms of the  spherical harmonic expansion/7(ct), Compute unnormalized associated  legendre polynomials and  derivatives via recursion relations/3(ct)
  st/1 -> Accumulate terms of the  spherical harmonic expansion/8(st), Compute unnormalized associated  legendre polynomials and  derivatives via recursion relations/2(st)
  dt/1 -> Time adjust the gauss coefficients/3(dt)
  event_time/1 -> Time adjust the gauss coefficients/Enable
  Constant/1 -> Sum1/2
  event_alt&lat/1 -> Compute unnormalized associated  legendre polynomials and  derivatives via recursion relations/Enable
  D4/1 -> For Iterator/1

== system Control_System_Library/Orbital Model/Subsystem/World Magnetic Model 2010/geomag/Convert from geodetic to  spherical coordinates/calculate ca ==
  alt : Inport
  r : Inport  Port=2
  d : Inport  Port=3
  Product11 : Product  Inputs=*/  SaturateOnIntegerOverflow=on  OutDataTypeStr=Inherit: Same as first input
  Sum8 : Sum  Inputs=|++  SaturateOnIntegerOverflow=on
  ca : Outport
  wires:
  Product11/1 -> ca/1
  d/1 -> Sum8/2
  alt/1 -> Sum8/1
  r/1 -> Product11/2
  Sum8/1 -> Product11/1

== system Control_System_Library/Orbital Model/Subsystem/World Magnetic Model 2010/geomag/Convert from geodetic to  spherical coordinates/calculate ct ==
  srlat : Inport
  q2 : Inport  Port=2
  crlat2 : Inport  Port=3
  srlat2 : Inport  Port=4
  Product3 : Product  SaturateOnIntegerOverflow=on  OutDataTypeStr=Inherit: Same as first input
  Product4 : Product  Inputs=*/  SaturateOnIntegerOverflow=on  OutDataTypeStr=Inherit: Same as first input
  Sum3 : Sum  Inputs=|++  SaturateOnIntegerOverflow=on
  sqrt : Sqrt  AlgorithmType=Newton-Raphson  SaturateOnIntegerOverflow=on
  ct : Outport
  wires:
  Product3/1 -> Sum3/2
  srlat2/1 -> Sum3/1
  q2/1 -> Product3/2
  crlat2/1 -> Product3/1
  Product4/1 -> ct/1
  srlat/1 -> Product4/1
  sqrt/1 -> Product4/2
  Sum3/1 -> sqrt/1

== system Control_System_Library/Orbital Model/Subsystem/World Magnetic Model 2010/geomag/Convert from geodetic to  spherical coordinates/calculate d ==
  a2 : Inport
  b2 : Inport  Port=2
  srlat2 : Inport  Port=3
  crlat2 : Inport  Port=4
  Product10 : Product  SaturateOnIntegerOverflow=on  OutDataTypeStr=Inherit: Same as first input
  Product9 : Product  SaturateOnIntegerOverflow=on  OutDataTypeStr=Inherit: Same as first input
  Sum7 : Sum  Inputs=++|  SaturateOnIntegerOverflow=on
  sqrt : Sqrt  AlgorithmType=Newton-Raphson  SaturateOnIntegerOverflow=on
  d : Outport
  wires:
  sqrt/1 -> d/1  "d"
  srlat2/1 -> Product10/2
  b2/1 -> Product10/1
  a2/1 -> Product9/2
  crlat2/1 -> Product9/1
  Product10/1 -> Sum7/2
  Product9/1 -> Sum7/1
  Sum7/1 -> sqrt/1

== system Control_System_Library/Orbital Model/Subsystem/World Magnetic Model 2010/geomag/Convert from geodetic to  spherical coordinates/calculate q ==
  a2 : Inport
  b2 : Inport  Port=2
  srlat2 : Inport  Port=3
  Product : Product  SaturateOnIntegerOverflow=on  OutDataTypeStr=Inherit: Same as first input
  Sum : Sum  Inputs=|-+  SaturateOnIntegerOverflow=on
  Sum1 : Sum  Inputs=|-+  SaturateOnIntegerOverflow=on
  sqrt : Sqrt  AlgorithmType=Newton-Raphson  SaturateOnIntegerOverflow=on
  q : Outport
  wires:
  b2/1 -> Sum1/1
  sqrt/1 -> q/1  "q"
  a2/1 -> Sum1/2, Sum/2
  Sum1/1 -> Product/2  "c2"
  srlat2/1 -> Product/1
  Sum/1 -> sqrt/1
  Product/1 -> Sum/1

== system Control_System_Library/Orbital Model/Subsystem/World Magnetic Model 2010/geomag/Convert from geodetic to  spherical coordinates/calculate q2 ==
  a2 : Inport
  b2 : Inport  Port=2
  q1 : Inport  Port=3
  Product1 : Product  SaturateOnIntegerOverflow=on  OutDataTypeStr=Inherit: Same as first input
  Product2 : Product  Inputs=**/  SaturateOnIntegerOverflow=on  OutDataTypeStr=Inherit: Same as first input
  Sum1 : Sum  Inputs=++|  SaturateOnIntegerOverflow=on
  Sum2 : Sum  Inputs=++|  SaturateOnIntegerOverflow=on
  q2 : Outport
  wires:
  Product1/1 -> Product2/3
  Product2/1 -> q2/1  "q2"
  b2/1 -> Sum1/2
  q1/1 -> Sum1/1, Sum2/2
  a2/1 -> Sum2/1
  Sum2/1 -> Product2/2, Product2/1
  Sum1/1 -> Product1/1, Product1/2

== system Control_System_Library/Orbital Model/Subsystem/World Magnetic Model 2010/geomag/Convert from geodetic to  spherical coordinates/calculate r2 ==
  q1 : Inport
  alt : Inport  Port=2
  q : Inport  Port=3
  a2 : Inport  Port=4
  b2 : Inport  Port=5
  srlat2 : Inport  Port=6
  Gain : Gain  Gain=2  SaturateOnIntegerOverflow=on  OutDataTypeStr=Inherit: Same as input  ParamDataTypeStr=Inherit: Same as input
  Product1 : Product  SaturateOnIntegerOverflow=on  OutDataTypeStr=Inherit: Same as first input
  Product6 : Product  SaturateOnIntegerOverflow=on  OutDataTypeStr=Inherit: Same as first input
  Product7 : Product  Inputs=*/  SaturateOnIntegerOverflow=on  OutDataTypeStr=Inherit: Same as first input
  Product8 : Product  SaturateOnIntegerOverflow=on  OutDataTypeStr=Inherit: Same as first input
  Sum5 : Sum  Inputs=+++  SaturateOnIntegerOverflow=on
  Sum6 : Sum  Inputs=|+-  SaturateOnIntegerOverflow=on
  Sum9 : Sum  Inputs=|+-  SaturateOnIntegerOverflow=on
  a4 : Product  SaturateOnIntegerOverflow=on  OutDataTypeStr=Inherit: Same as first input
  b4 : Product  SaturateOnIntegerOverflow=on  OutDataTypeStr=Inherit: Same as first input
  r2 : Outport
  wires:
  Product1/1 -> Product7/2
  b2/1 -> b4/1, b4/2
  b4/1 -> Sum9/2
  Sum5/1 -> r2/1  "r2"
  srlat2/1 -> Product8/2
  a2/1 -> a4/2, a4/1
  alt/1 -> Product6/1, Product6/2
  q/1 -> Product1/1, Product1/2
  q1/1 -> Gain/1
  a4/1 -> Sum6/1, Sum9/1
  Sum9/1 -> Product8/1  "c4"
  Product8/1 -> Sum6/2
  Sum6/1 -> Product7/1
  Product7/1 -> Sum5/3
  Gain/1 -> Sum5/1
  Product6/1 -> Sum5/2

== system Control_System_Library/Orbital Model/Subsystem/World Magnetic Model 2010/geomag/Convert from geodetic to  spherical coordinates/calculate sa ==
  a2 : Inport
  b2 : Inport  Port=2
  r : Inport  Port=3
  d : Inport  Port=4
  crlat : Inport  Port=5
  srlat : Inport  Port=6
  Product1 : Product  SaturateOnIntegerOverflow=on  OutDataTypeStr=Inherit: Same as first input
  Product12 : Product  Inputs=*/**  SaturateOnIntegerOverflow=on  OutDataTypeStr=Inherit: Same as first input
  Sum1 : Sum  Inputs=|-+  SaturateOnIntegerOverflow=on
  sa : Outport
  wires:
  Product1/1 -> Product12/2
  crlat/1 -> Product12/3
  srlat/1 -> Product12/4
  Product12/1 -> sa/1
  a2/1 -> Sum1/2
  b2/1 -> Sum1/1
  d/1 -> Product1/2
  r/1 -> Product1/1
  Sum1/1 -> Product12/1  "c2"

== system Control_System_Library/Orbital Model/Subsystem/World Magnetic Model 2010/geomag/Convert from geodetic to  spherical coordinates/calculate st ==
  ct : Inport
  Constant : Constant  OutDataTypeStr=Inherit: Inherit via back propagation
  Product5 : Product  SaturateOnIntegerOverflow=on  OutDataTypeStr=Inherit: Same as first input
  Sum4 : Sum  Inputs=|-+  SaturateOnIntegerOverflow=on
  sqrt : Sqrt  AlgorithmType=Newton-Raphson  SaturateOnIntegerOverflow=on
  st : Outport
  wires:
  sqrt/1 -> st/1
  ct/1 -> Product5/2, Product5/1
  Constant/1 -> Sum4/2
  Sum4/1 -> sqrt/1
  Product5/1 -> Sum4/1

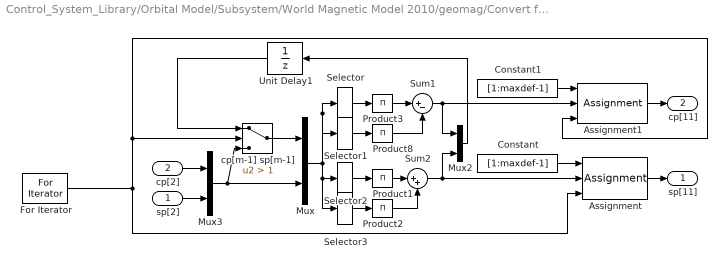
== system Control_System_Library/Orbital Model/Subsystem/World Magnetic Model 2010/geomag/Convert from geodetic to  spherical coordinates /For Iterator Subsystem ==
  sp[2] : Inport
  cp[2] : Inport  Port=2
  Assignment : Assignment  DiagnosticForDimensions=Error  IndexOptions=Index vector (port)  Indices=1  OutputSizes=[1 1]
  Assignment1 : Assignment  DiagnosticForDimensions=Error  IndexOptions=Index vector (port)  Indices=1  OutputSizes=[1 1]
  Constant : Constant  Value=[1:maxdef-1]  OutDataTypeStr=Inherit: Inherit via back propagation
  Constant1 : Constant  Value=[1:maxdef-1]  OutDataTypeStr=Inherit: Inherit via back propagation
  For Iterator : ForIterator  IterationLimit=maxdef-1  IterationVariableDataType=double
  Mux : Mux  Inputs=[2 2]
  Mux2 : Mux  Inputs=2
  Mux3 : Mux  Inputs=2
  Product{1..3,8} (4 alike) : Product  Inputs=1  SaturateOnIntegerOverflow=on  OutDataTypeStr=Inherit: Same as first input
  Selector : Selector  InputPortWidth=4  IndexOptions=Index vector (dialog)  Indices=[1 3]  OutputSizes=1
  Selector1 : Selector  InputPortWidth=4  IndexOptions=Index vector (dialog)  Indices=[2 4]  OutputSizes=1
  Selector2 : Selector  InputPortWidth=4  IndexOptions=Index vector (dialog)  Indices=[1 4]  OutputSizes=1
  Selector3 : Selector  InputPortWidth=4  IndexOptions=Index vector (dialog)  Indices=[2 3]  OutputSizes=1
  Sum1 : Sum  Inputs=|+-  SaturateOnIntegerOverflow=on
  Sum2 : Sum  Inputs=|++  SaturateOnIntegerOverflow=on
  Unit Delay1 : UnitDelay  SampleTime=-1
  cp[m-1] sp[m-1] : Switch  Criteria=u2 > Threshold  Threshold=1  SaturateOnIntegerOverflow=on
  sp[11] : Outport
  cp[11] : Outport  Port=2
  wires:
  Mux3/1 -> cp[m-1] sp[m-1]/3, Mux/2
  Mux2/1 -> Unit Delay1/1
  Selector3/1 -> Product2/1
  Selector2/1 -> Product1/1
  Selector1/1 -> Product8/1
  Mux/1 -> Selector2/1, Selector3/1, Selector1/1, Selector/1
  Selector/1 -> Product3/1
  cp[m-1] sp[m-1]/1 -> Mux/1
  Constant1/1 -> Assignment1/1
  For Iterator/1 -> Assignment/3, cp[m-1] sp[m-1]/2, Assignment1/3
  sp[2]/1 -> Mux3/2
  cp[2]/1 -> Mux3/1
  Assignment1/1 -> cp[11]/1
  Product3/1 -> Sum1/1
  Product8/1 -> Sum1/2
  Product1/1 -> Sum2/1
  Product2/1 -> Sum2/2
  Sum2/1 -> Mux2/2, Assignment/2
  Sum1/1 -> Mux2/1, Assignment1/2
  Unit Delay1/1 -> cp[m-1] sp[m-1]/1
  Assignment/1 -> sp[11]/1
  Constant/1 -> Assignment/1

== system Control_System_Library/Orbital Model/Subsystem/World Magnetic Model 2010/geomag/Rotate magnetic vector components  to geodetic from spherical and  compute declination, inclination  and total intensity/Calculate bx ==
  ca : Inport
  sa : Inport  Port=2
  bt : Inport  Port=3
  br : Inport  Port=4
  Product1 : Product  SaturateOnIntegerOverflow=on  OutDataTypeStr=Inherit: Same as first input
  Product4 : Product  SaturateOnIntegerOverflow=on  OutDataTypeStr=Inherit: Same as first input
  Sum1 : Sum  Inputs=|--  SaturateOnIntegerOverflow=on
  bx : Outport
  wires:
  sa/1 -> Product4/2
  Sum1/1 -> bx/1  "bx"
  ca/1 -> Product1/1
  br/1 -> Product4/1
  bt/1 -> Product1/2
  Product4/1 -> Sum1/2
  Product1/1 -> Sum1/1

== system Control_System_Library/Orbital Model/Subsystem/World Magnetic Model 2010/geomag/Rotate magnetic vector components  to geodetic from spherical and  compute declination, inclination  and total intensity/Calculate by ==
  bp : Inport
  st : Inport  Port=2
  bpp : Inport  Port=3
  Product : Product  Inputs=*/  SaturateOnIntegerOverflow=on  OutDataTypeStr=Inherit: Same as first input
  Switch : Switch  Criteria=u2 ~= 0  SaturateOnIntegerOverflow=on
  by : Outport
  wires:
  bpp/1 -> Switch/3
  Switch/1 -> by/1  "by"
  bp/1 -> Product/1
  Product/1 -> Switch/1
  st/1 -> Switch/2, Product/2

== system Control_System_Library/Orbital Model/Subsystem/World Magnetic Model 2010/geomag/Rotate magnetic vector components  to geodetic from spherical and  compute declination, inclination  and total intensity/Calculate bz ==
  ca : Inport
  sa : Inport  Port=2
  bt : Inport  Port=3
  br : Inport  Port=4
  Product1 : Product  SaturateOnIntegerOverflow=on  OutDataTypeStr=Inherit: Same as first input
  Product4 : Product  SaturateOnIntegerOverflow=on  OutDataTypeStr=Inherit: Same as first input
  Sum1 : Sum  Inputs=|+-  SaturateOnIntegerOverflow=on
  bz : Outport
  wires:
  Product1/1 -> Sum1/1
  Product4/1 -> Sum1/2
  bt/1 -> Product1/2
  br/1 -> Product4/1
  sa/1 -> Product1/1
  Sum1/1 -> bz/1  "bz"
  ca/1 -> Product4/2
